simulink model "aizawa_sim"  (R2021a)
settings: Solver=VariableStepAuto  StartTime=0.0  StopTime=tFinal  MaxStep=tMaxStep  RelTol=1e-3
values from neighbouring files (symbols this model uses):
  a = tic    [aizawa_system_visualization.m]
  b = toc(a)    [aizawa_system_visualization.m]
undefined symbols (not defined in the file or in its folder): c, d, f, x0
settings Model: Creator=toure  LastModifiedBy=toure

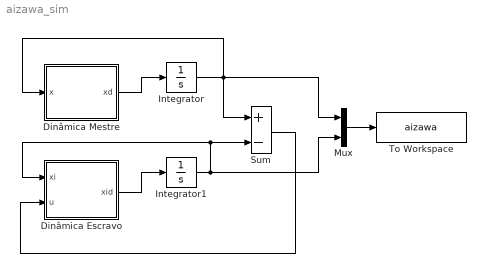
== system aizawa_sim ==
  Dinâmica Escravo : MATLAB Function  TreatAsAtomicUnit=on
  Dinâmica Mestre : MATLAB Function  TreatAsAtomicUnit=on
  Integrator : Integrator  InitialCondition=x0
  Integrator1 : Integrator  InitialCondition=x0+.001
  Mux : Mux  Inputs=2
  Sum : Sum  Inputs=+-
  To Workspace : ToWorkspace  VariableName=aizawa  SaveFormat=Timeseries  SampleTime=-1
  wires:
  Dinâmica Escravo/1(xid) -> Integrator1/1
  Dinâmica Mestre/1(xd) -> Integrator/1
  Integrator/1 -> Mux/1, Sum/1, Dinâmica Mestre/1(x)
  Integrator1/1 -> Mux/2, Dinâmica Escravo/1(xi), Sum/2
  Mux/1 -> To Workspace/1
  Sum/1 -> Dinâmica Escravo/2(u)

== matlab function aizawa_sim/Dinâmica Escravo ==
  data: xi input; u input; xid output; a parameter; b parameter; c parameter; d parameter; e parameter; f parameter
function xid = fcn(xi, u, a, b, c, d, e, f)

xid = [(xi(3) - b)*xi(1) - d*xi(2) + u(1)
        d*xi(1) + (xi(3) - b)*xi(2) + u(2)
        c + a*xi(3) - (1/3)*xi(3)^3 - (xi(1)^2 + xi(2)^2)*(1 + e*xi(3)) + f*xi(3)*xi(1)^3 + u(3)];
end

== matlab function aizawa_sim/Dinâmica Mestre ==
  data: x input; xd output; a parameter; b parameter; c parameter; d parameter; e parameter; f parameter
function xd = fcn(x, a, b, c, d, e, f)

xd = [(x(3) - b)*x(1) - d*x(2)
       d*x(1) + (x(3) - b)*x(2)
       c + a*x(3) - (1/3)*x(3)^3 - (x(1)^2 + x(2)^2)*(1 + e*x(3)) + f*x(3)*x(1)^3];
end
